simulink model "data_view"  (Simulink 7.6)
settings: Solver=FixedStepDiscrete  StartTime=0.0  StopTime=20000  FixedStep=1  RelTol=1e-3
settings Model: Creator=jordan  LastModifiedBy=jordan

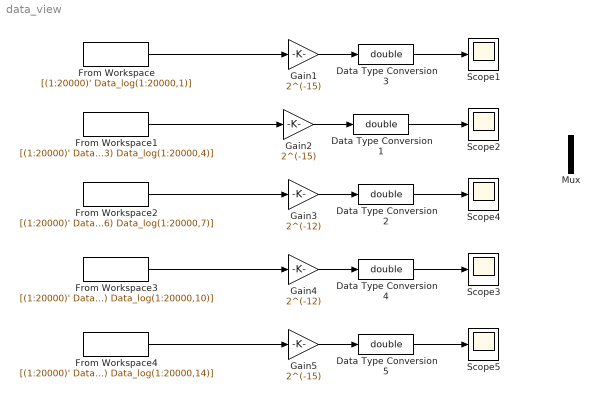
== system data_view ==
  Data Type Conversion{1..5} (5 alike) : DataTypeConversion  OutDataTypeStr=double  SaturateOnIntegerOverflow=on
  From Workspace : FromWorkspace  VariableName=[(1:20000)' Data_log(1:20000,1)]  SampleTime=1  Interpolate=off  OutputAfterFinalValue=Setting to zero
  From Workspace1 : FromWorkspace  VariableName=[(1:20000)' Data_log(1:20000,2) Data_log(1:20000,3) Data_log(1:20000,4)]  SampleTime=1  Interpolate=off  OutputAfterFinalValue=Setting to zero
  From Workspace2 : FromWorkspace  VariableName=[(1:20000)' Data_log(1:20000,5) Data_log(1:20000,6) Data_log(1:20000,7)]  SampleTime=1  Interpolate=off  OutputAfterFinalValue=Setting to zero
  From Workspace3 : FromWorkspace  VariableName=[(1:20000)' Data_log(1:20000,8) Data_log(1:20000,9) Data_log(1:20000,10)]  SampleTime=1  Interpolate=off  OutputAfterFinalValue=Setting to zero
  From Workspace4 : FromWorkspace  VariableName=[(1:20000)' Data_log(1:20000,11) Data_log(1:20000,12) Data_log(1:20000,13) Data_log(1:20000,14)]  SampleTime=1  Interpolate=off  OutputAfterFinalValue=Setting to zero
  Gain1 : Gain  Gain=2^(-15)  OutDataTypeStr=fixdt(1,16,15)
  Gain2 : Gain  Gain=2^(-15)  OutDataTypeStr=fixdt(1,16,15)
  Gain3 : Gain  Gain=2^(-12)  OutDataTypeStr=fixdt(1,16,12)
  Gain4 : Gain  Gain=2^(-12)  OutDataTypeStr=fixdt(1,16,12)
  Gain5 : Gain  Gain=2^(-15)  OutDataTypeStr=fixdt(1,16,15)
  Mux : Mux  Inputs=3
  Scope{1..5} (5 alike) : Scope
      Scope1 settings: TimeRange=4000  YMin=0  YMax=0.35
      Scope2 settings: TimeRange=4000  YMin=0  YMax=0.35  MaxDataPoints=50000
      Scope3 settings: TimeRange=4000  YMin=0  YMax=0.35  SaveName=ScopeData3  MaxDataPoints=50000
      Scope4 settings: TimeRange=4000  YMin=0  YMax=0.35  SaveName=ScopeData2  MaxDataPoints=50000
      Scope5 settings: TimeRange=4000  YMin=0  YMax=0.35  SaveName=ScopeData4  MaxDataPoints=50000
  wires:
  Gain1/1 -> Data Type Conversion3/1
  From Workspace/1 -> Gain1/1
  Gain2/1 -> Data Type Conversion1/1
  From Workspace1/1 -> Gain2/1
  Gain3/1 -> Data Type Conversion2/1
  From Workspace2/1 -> Gain3/1
  Data Type Conversion1/1 -> Scope2/1
  Data Type Conversion3/1 -> Scope1/1
  Data Type Conversion2/1 -> Scope4/1
  Gain4/1 -> Data Type Conversion4/1
  From Workspace3/1 -> Gain4/1
  Data Type Conversion4/1 -> Scope3/1
  Gain5/1 -> Data Type Conversion5/1
  From Workspace4/1 -> Gain5/1
  Data Type Conversion5/1 -> Scope5/1
